simulink model "mod_torque_y_obvservador_de_velocidad"  (R2016a)
settings: Solver=VariableStepAuto  StartTime=0.0  StopTime=10.0  RelTol=1e-3
values from neighbouring files (symbols this model uses):
  beq = (bm+bl/r^2)    (= 1.5637748692e-05)    [parametros.m]    (also in planificador_de_trayectoria.m)
  Cts = 1.091    [parametros.m]
  Jeq = (Jm+Jl/r^2)    (= 6.92649215207e-06)    [parametros.m]    (also in planificador_de_trayectoria.m)
  K_tita = 6397.3    [parametros.m]
  Kw = 1.0223e7    (= 10223000)    [parametros.m]
  lambda_m = 0.01546    [parametros.m]
  Ld = 6.6e-3    (= 0.0066)    [parametros.m]
  Lls = 0.8e-3    (= 0.0008)    [parametros.m]
  Lq = 5.8e-3    (= 0.0058)    [parametros.m]
  Pp = 3    [parametros.m]
  r = 314.3008    [parametros.m]    (also in planificador_de_trayectoria.m)
  Rp_d = 5000*Ld    (= 33)    [parametros.m]
  Rp_q = 5000*Lq    (= 29)    [parametros.m]
  Rs = 1.02    [parametros.m]
  Rs_amb = 55    [parametros.m]
libraries: powerlib_meascontrol x4
settings Model: Creator=Jere  LastModifiedBy=Jere
settings GRTTargetCC: GeneratePreprocessorConditionals=Use local settings

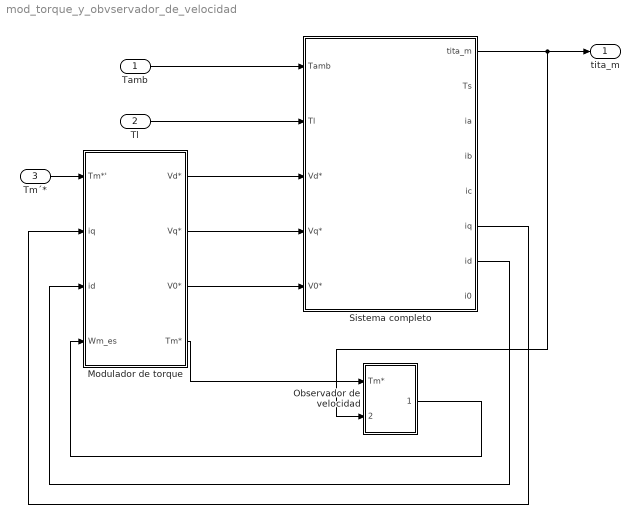
== system mod_torque_y_obvservador_de_velocidad ==
  Tamb : Inport
  Tl : Inport  Port=2
  Tm´* : Inport  Port=3
  Modulador de torque : Subsystem
  Observador de velocidad : Subsystem
  Sistema completo : Subsystem
  tita_m : Outport
  wires:
  Tamb/1 -> Sistema completo/1(Tamb)
  Tl/1 -> Sistema completo/2(Tl)
  Sistema completo/1(tita_m) -> Observador de velocidad/2(tita_m), tita_m/1
  Modulador de torque/1(Vd*) -> Sistema completo/3(Vd*)
  Modulador de torque/2(Vq*) -> Sistema completo/4(Vq*)
  Modulador de torque/3(V0*) -> Sistema completo/5(V0*)
  Modulador de torque/4(Tm*) -> Observador de velocidad/1(Tm*)
  Observador de velocidad/1(Wm_es) -> Modulador de torque/4(Wm_es)
  Sistema completo/6(iq) -> Modulador de torque/2(iq)
  Sistema completo/7(id) -> Modulador de torque/3(id)
  Tm´*/1 -> Modulador de torque/1(Tm*')

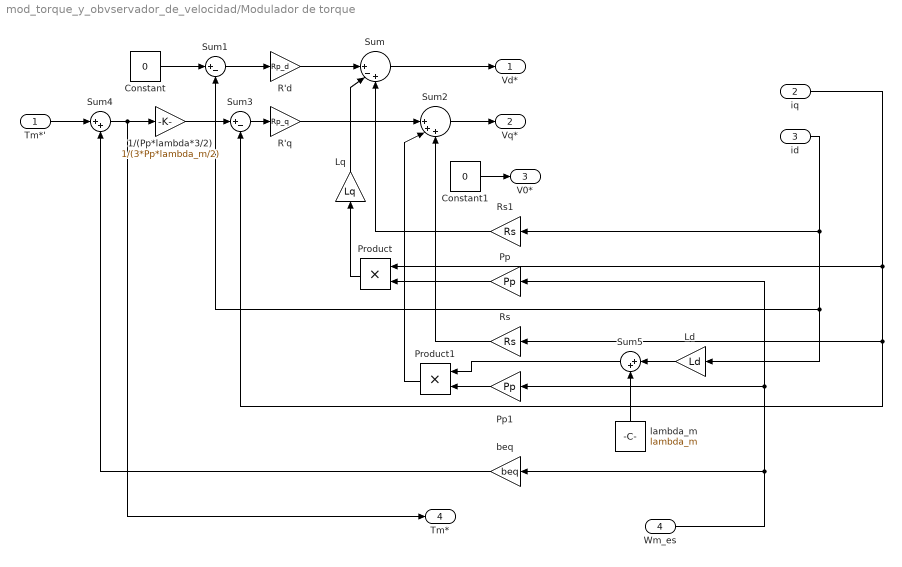
== system mod_torque_y_obvservador_de_velocidad/Modulador de torque ==
  Tm*' : Inport
  iq : Inport  Port=2
  id : Inport  Port=3
  Wm_es : Inport  Port=4
  1/(Pp*lambda*3/2) : Gain  Gain=1/(3*Pp*lambda_m/2)
  Constant : Constant  Value=0
  Constant1 : Constant  Value=0
  Ld : Gain  Gain=Ld
  Lq : Gain  Gain=Lq
  Pp : Gain  Gain=Pp
  Pp1 : Gain  Gain=Pp
  Product : Product
  Product1 : Product
  R'd : Gain  Gain=Rp_d
  R'q : Gain  Gain=Rp_q
  Rs : Gain  Gain=Rs
  Rs1 : Gain  Gain=Rs
  Sum : Sum  Inputs=||+-+
  Sum1 : Sum  Inputs=|+-
  Sum2 : Sum  Inputs=||+++
  Sum3 : Sum  Inputs=|+-
  Sum4 : Sum  Inputs=|++
  Sum5 : Sum  Inputs=|++
  beq : Gain  Gain=beq
  lambda_m : Constant  Value=lambda_m
  Vd* : Outport
  Vq* : Outport  Port=2
  V0* : Outport  Port=3
  Tm* : Outport  Port=4
  wires:
  Product1/1 -> Sum2/2
  Sum/1 -> Vd*/1
  Sum2/1 -> Vq*/1
  id/1 -> Ld/1, Sum1/2, Rs1/1
  Wm_es/1 -> Pp/1, Pp1/1, beq/1
  lambda_m/1 -> Sum5/2
  beq/1 -> Sum4/2
  Pp1/1 -> Product1/2
  Constant/1 -> Sum1/1
  Ld/1 -> Sum5/1
  iq/1 -> Sum3/2, Rs/1, Product/1
  Rs1/1 -> Sum/3
  Sum5/1 -> Product1/1
  Lq/1 -> Sum/2
  Product/1 -> Lq/1
  Tm*'/1 -> Sum4/1
  Pp/1 -> Product/2
  Sum1/1 -> R'd/1
  R'd/1 -> Sum/1
  Sum3/1 -> R'q/1
  R'q/1 -> Sum2/1
  Constant1/1 -> V0*/1
  Rs/1 -> Sum2/3
  1/(Pp*lambda*3/2)/1 -> Sum3/1
  Sum4/1 -> Tm*/1, 1/(Pp*lambda*3/2)/1

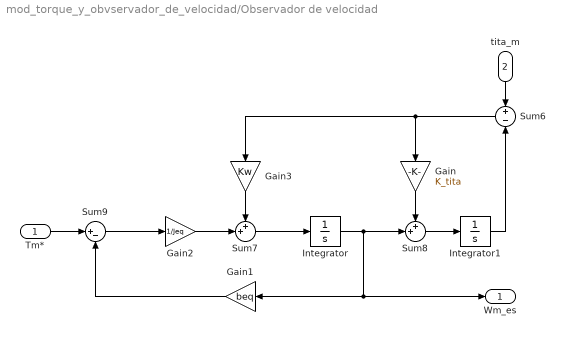
== system mod_torque_y_obvservador_de_velocidad/Observador de velocidad ==
  Tm* : Inport
  tita_m : Inport  Port=2
  Gain : Gain  Gain=K_tita
  Gain1 : Gain  Gain=beq
  Gain2 : Gain  Gain=1/Jeq
  Gain3 : Gain  Gain=Kw
  Integrator : Integrator
  Integrator1 : Integrator
  Sum6 : Sum  Inputs=+|-
  Sum7 : Sum  Inputs=++|
  Sum8 : Sum  Inputs=++|
  Sum9 : Sum  Inputs=|+-
  Wm_es : Outport
  wires:
  Gain/1 -> Sum8/1
  Sum8/1 -> Integrator1/1
  Integrator/1 -> Wm_es/1, Gain1/1, Sum8/2
  Sum7/1 -> Integrator/1
  Tm*/1 -> Sum9/1
  Integrator1/1 -> Sum6/2
  Gain3/1 -> Sum7/1
  Gain1/1 -> Sum9/2
  Sum9/1 -> Gain2/1
  Gain2/1 -> Sum7/2
  Sum6/1 -> Gain3/1, Gain/1
  tita_m/1 -> Sum6/1

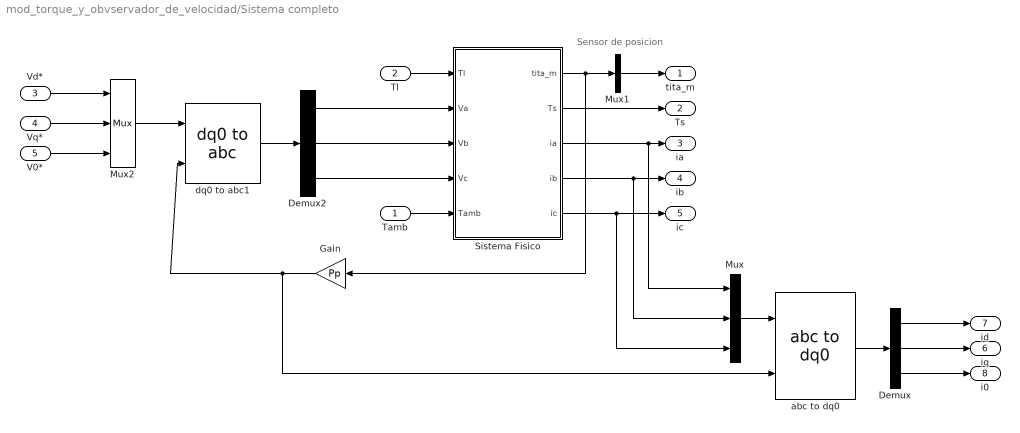
== system mod_torque_y_obvservador_de_velocidad/Sistema completo ==
  note: Sensor de posicion
  Tamb : Inport
  Tl : Inport  Port=2
  Vd* : Inport  Port=3
  Vq* : Inport  Port=4
  V0* : Inport  Port=5
  Demux : Demux  Outputs=3
  Demux2 : Demux  Outputs=3
  Gain : Gain  Gain=Pp
  Mux : Mux  Inputs=3
  Mux1 : Mux  Inputs=1
  Mux2 : Mux  Inputs=3
  Sistema Fisico : Subsystem
  abc to dq0 : powerlib_meascontrol/Transformations/abc to dq0  Alignment=90 degrees behind phase A axis
  dq0 to abc1 : powerlib_meascontrol/Transformations/dq0 to abc  Alignment=90 degrees behind phase A axis
  tita_m : Outport
  Ts : Outport  Port=2
  ia : Outport  Port=3
  ib : Outport  Port=4
  ic : Outport  Port=5
  iq : Outport  Port=6
  id : Outport  Port=7
  i0 : Outport  Port=8
  wires:
  Mux2/1 -> dq0 to abc1/1
  dq0 to abc1/1 -> Demux2/1
  Vd*/1 -> Mux2/1
  Vq*/1 -> Mux2/2
  V0*/1 -> Mux2/3
  Tl/1 -> Sistema Fisico/1(Tl)
  Demux2/1 -> Sistema Fisico/2(Va)
  Demux2/2 -> Sistema Fisico/3(Vb)
  Demux2/3 -> Sistema Fisico/4(Vc)
  Tamb/1 -> Sistema Fisico/5(Tamb)
  Sistema Fisico/1(tita_m) -> Gain/1, Mux1/1
  Sistema Fisico/2(Ts) -> Ts/1
  Mux/1 -> abc to dq0/1
  abc to dq0/1 -> Demux/1
  Sistema Fisico/5(ic) -> ic/1, Mux/3
  Sistema Fisico/3(ia) -> ia/1, Mux/1
  Sistema Fisico/4(ib) -> ib/1, Mux/2
  Gain/1 -> abc to dq0/2, dq0 to abc1/2
  Demux/3 -> i0/1
  Demux/1 -> id/1
  Demux/2 -> iq/1
  Mux1/1 -> tita_m/1

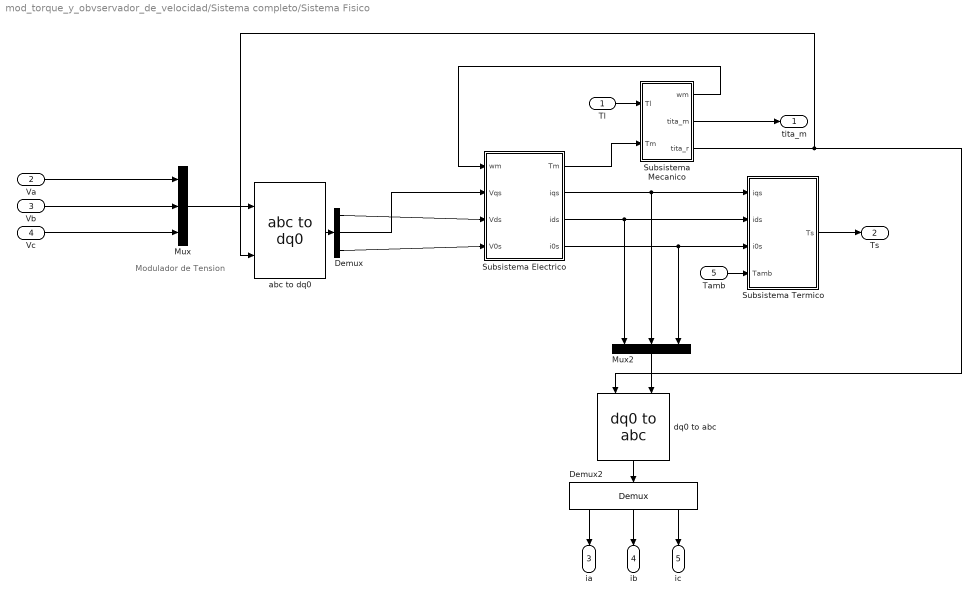
== system mod_torque_y_obvservador_de_velocidad/Sistema completo/Sistema Fisico ==
  note: Modulador de Tension
  Tl : Inport
  Va : Inport  Port=2
  Vb : Inport  Port=3
  Vc : Inport  Port=4
  Tamb : Inport  Port=5
  Demux : Demux  Outputs=3
  Demux2 : Demux  Outputs=3
  Mux : Mux  Inputs=3
  Mux2 : Mux  Inputs=3
  Subsistema Electrico : Subsystem
  Subsistema Mecanico : Subsystem
  Subsistema Termico : Subsystem
  abc to dq0 : powerlib_meascontrol/Transformations/abc to dq0  Alignment=90 degrees behind phase A axis
  dq0 to abc : powerlib_meascontrol/Transformations/dq0 to abc  Alignment=90 degrees behind phase A axis
  tita_m : Outport
  Ts : Outport  Port=2
  ia : Outport  Port=3
  ib : Outport  Port=4
  ic : Outport  Port=5
  wires:
  dq0 to abc/1 -> Demux2/1
  Mux/1 -> abc to dq0/1
  Subsistema Termico/1(Ts) -> Ts/1
  Tamb/1 -> Subsistema Termico/4(Tamb)
  Subsistema Mecanico/1(wm) -> Subsistema Electrico/1(wm)
  Tl/1 -> Subsistema Mecanico/1(Tl)
  Demux/1 -> Subsistema Electrico/3(Vds)
  Demux/3 -> Subsistema Electrico/4(V0s)
  Subsistema Electrico/1(Tm) -> Subsistema Mecanico/2(Tm)
  Subsistema Electrico/2(iqs) -> Mux2/2, Subsistema Termico/1(iqs)
  Subsistema Electrico/3(ids) -> Mux2/1, Subsistema Termico/2(ids)
  Subsistema Electrico/4(i0s) -> Mux2/3, Subsistema Termico/3(i0s)
  Demux/2 -> Subsistema Electrico/2(Vqs)
  Demux2/2 -> ib/1
  abc to dq0/1 -> Demux/1
  Demux2/1 -> ia/1
  Mux2/1 -> dq0 to abc/1
  Demux2/3 -> ic/1
  Vc/1 -> Mux/3
  Va/1 -> Mux/1
  Subsistema Mecanico/3(tita_r) -> abc to dq0/2, dq0 to abc/2
  Vb/1 -> Mux/2
  Subsistema Mecanico/2(tita_m) -> tita_m/1

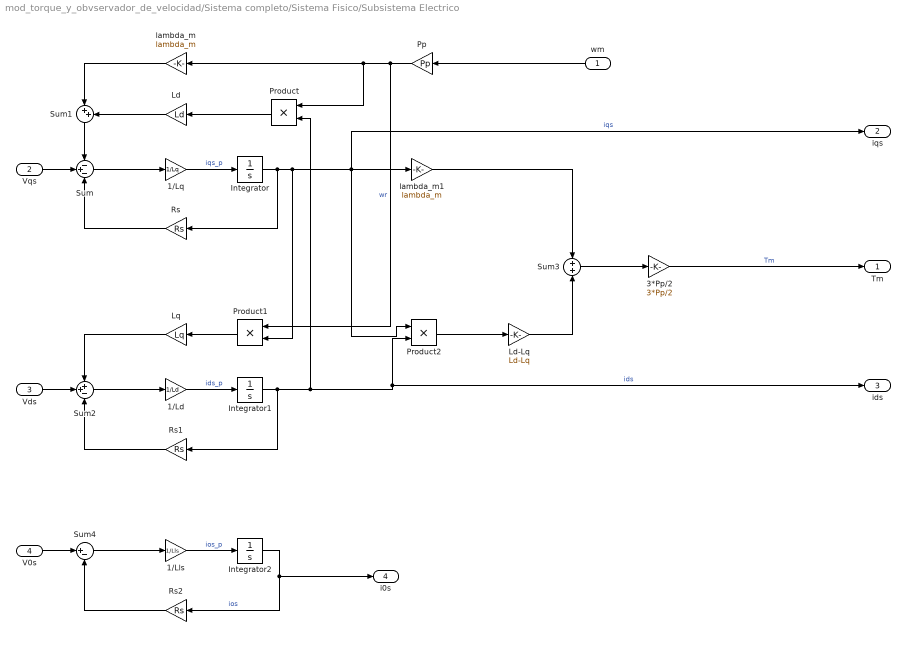
== system mod_torque_y_obvservador_de_velocidad/Sistema completo/Sistema Fisico/Subsistema Electrico ==
  wm : Inport
  Vqs : Inport  Port=2
  Vds : Inport  Port=3
  V0s : Inport  Port=4
  1/Ld : Gain  Gain=1/Ld
  1/Lls : Gain  Gain=1/Lls
  1/Lq : Gain  Gain=1/Lq
  3*Pp/2 : Gain  Gain=3*Pp/2
  Integrator : Integrator
  Integrator1 : Integrator
  Integrator2 : Integrator
  Ld : Gain  Gain=Ld
  Ld-Lq : Gain  Gain=Ld-Lq
  Lq : Gain  Gain=Lq
  Pp : Gain  Gain=Pp
  Product : Product
  Product1 : Product
  Product2 : Product
  Rs : Gain  Gain=Rs
  Rs1 : Gain  Gain=Rs
  Rs2 : Gain  Gain=Rs
  Sum : Sum  Inputs=-+-
  Sum1 : Sum  Inputs=|++
  Sum2 : Sum  Inputs=++-
  Sum3 : Sum
  Sum4 : Sum  Inputs=|+-
  lambda_m : Gain  Gain=lambda_m
  lambda_m1 : Gain  Gain=lambda_m
  Tm : Outport
  iqs : Outport  Port=2
  ids : Outport  Port=3
  i0s : Outport  Port=4
  wires:
  wm/1 -> Pp/1
  3*Pp/2/1 -> Tm/1  "Tm"
  Sum1/1 -> Sum/1
  lambda_m1/1 -> Sum3/1
  Sum/1 -> 1/Lq/1
  Vds/1 -> Sum2/2
  Integrator2/1 -> i0s/1, Rs2/1  "ios"
  Rs1/1 -> Sum2/3
  Integrator1/1 -> Product/2, Product2/2, ids/1, Rs1/1  "ids"
  Integrator/1 -> Product1/2, Product2/1, iqs/1, lambda_m1/1, Rs/1  "iqs"
  Sum3/1 -> 3*Pp/2/1
  Ld/1 -> Sum1/2
  Product1/1 -> Lq/1
  Product2/1 -> Ld-Lq/1
  Ld-Lq/1 -> Sum3/2
  1/Ld/1 -> Integrator1/1  "ids_p"
  Lq/1 -> Sum2/1
  V0s/1 -> Sum4/1
  Sum2/1 -> 1/Ld/1
  1/Lq/1 -> Integrator/1  "iqs_p"
  Vqs/1 -> Sum/2
  Pp/1 -> Product1/1, Product/1, lambda_m/1  "wr"
  lambda_m/1 -> Sum1/1
  Rs/1 -> Sum/3
  1/Lls/1 -> Integrator2/1  "ios_p"
  Rs2/1 -> Sum4/2
  Product/1 -> Ld/1
  Sum4/1 -> 1/Lls/1

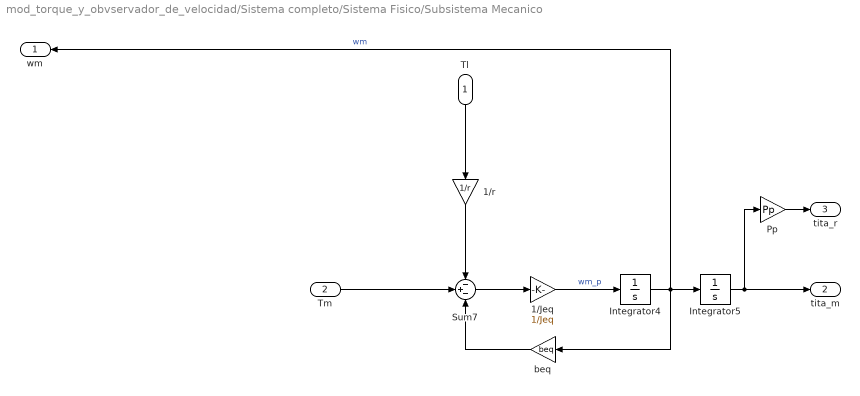
== system mod_torque_y_obvservador_de_velocidad/Sistema completo/Sistema Fisico/Subsistema Mecanico ==
  Tl : Inport
  Tm : Inport  Port=2
  1/Jeq : Gain  Gain=1/Jeq
  1/r : Gain  Gain=1/r
  Integrator4 : Integrator
  Integrator5 : Integrator
  Pp : Gain  Gain=Pp
  Sum7 : Sum  Inputs=-+-
  beq : Gain  Gain=beq
  wm : Outport
  tita_m : Outport  Port=2
  tita_r : Outport  Port=3
  wires:
  beq/1 -> Sum7/3
  Sum7/1 -> 1/Jeq/1
  Tl/1 -> 1/r/1
  1/Jeq/1 -> Integrator4/1  "wm_p"
  Integrator5/1 -> Pp/1, tita_m/1
  Tm/1 -> Sum7/2
  Integrator4/1 -> wm/1, Integrator5/1, beq/1  "wm"
  1/r/1 -> Sum7/1
  Pp/1 -> tita_r/1

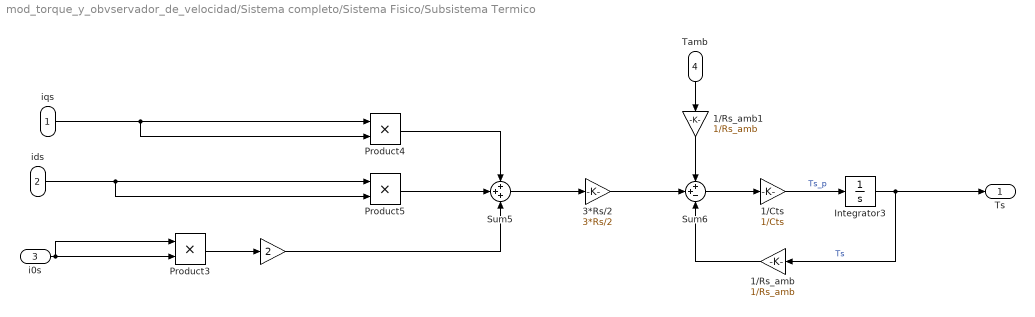
== system mod_torque_y_obvservador_de_velocidad/Sistema completo/Sistema Fisico/Subsistema Termico ==
  iqs : Inport
  ids : Inport  Port=2
  i0s : Inport  Port=3
  Tamb : Inport  Port=4
  " " : Gain  Gain=2
  1/Cts : Gain  Gain=1/Cts
  1/Rs_amb : Gain  Gain=1/Rs_amb
  1/Rs_amb1 : Gain  Gain=1/Rs_amb
  3*Rs/2 : Gain  Gain=3*Rs/2
  Integrator3 : Integrator
  Product3 : Product
  Product4 : Product
  Product5 : Product
  Sum5 : Sum  Inputs=+++
  Sum6 : Sum  Inputs=++-
  Ts : Outport
  wires:
  iqs/1 -> Product4/2, Product4/1
  i0s/1 -> Product3/1, Product3/2
  ids/1 -> Product5/2, Product5/1
  Product3/1 -> " "/1
  " "/1 -> Sum5/3
  Sum6/1 -> 1/Cts/1
  Product4/1 -> Sum5/1
  3*Rs/2/1 -> Sum6/2
  Tamb/1 -> 1/Rs_amb1/1
  Product5/1 -> Sum5/2
  1/Rs_amb/1 -> Sum6/3
  Sum5/1 -> 3*Rs/2/1
  1/Cts/1 -> Integrator3/1  "Ts_p"
  Integrator3/1 -> Ts/1, 1/Rs_amb/1  "Ts"
  1/Rs_amb1/1 -> Sum6/1
